simulink model "PIDnANNsim"  (R2021a)
settings: Solver=ode45  StartTime=0.0  StopTime=60  RelTol=1e-3  AbsTol=1e-6
undefined symbols (not defined in the file or in its folder): now, sfunxy2
libraries: neural x1, pid_lib x1
settings Model: ExtModeTrigMode=oneshot  ExtModeArmWhenConnect=off  TunableVars=prueba  TunableVarsStorageClass=Auto  Creator=The MathWorks, Inc.  LastModifiedBy=914487352
settings SolverCC: AutoScaleAbsTol=off  AlgebraicLoopSolver=TrustRegion
settings DataIOCC: SaveFormat=Array  SaveOutput=off  ReturnWorkspaceOutputs=off  SignalLoggingName=sigsOut
settings OptimizationCC: BooleanDataType=off  DefaultParameterBehavior=Inlined  ExpressionDepthLimit=2147483647  InitFltsAndDblsToZero=on  LifeSpan=inf
settings DebuggingCC: SaveWithParameterizedLinksMsg=none  UnderspecifiedInitializationDetection=Classic  MergeDetectMultiDrivingBlocksExec=none  SignalResolutionControl=TryResolveAllWithWarning  MultiTaskDSMMsg=warning  MultiTaskCondExecSysMsg=none  FcnCallInpInsideContextMsg=warning  StateNameClashWarn=warning  SFUnexpectedBacktrackingDiag=warning  SFNoUnconditionalDefaultTransitionDiag=warning  SFExecutionAtInitializationDiag=none  SFMachineParentedDataDiag=warning  ArithmeticOperatorsInVariantConditions=warning
settings HardwareCC: ProdBitPerPointer=32  ProdBitPerSizeT=32  ProdBitPerPtrDiffT=32  ProdLargestAtomicFloat=None  ProdIntDivRoundTo=Undefined  ProdEndianess=Unspecified  ProdWordSize=32  ProdHWDeviceType=32-bit Generic  TargetUnknown=on
settings ModelReferenceCC: PropagateSignalLabelsOutOfModel=off
settings SFSimCC: SimUseLocalCustomCode=off  CustomCodeUndefinedFunction=UseInterfaceOnly
settings RTWCC: TemplateMakefile=grt_vc.tmf  RTWUseLocalCustomCode=off
settings CodeAppCC: StateflowObjectComments=on
settings GRTTargetCC: TargetFcnLib=ansi_tfl_tmw.mat  TargetLangStandard=C89/C90 (ANSI)  CombineOutputUpdateFcns=off  GRTInterface=on
settings ConfigComp: CovMetricSettings=dw  CovSaveCumulativeToWorkspaceVar=on  CovSaveSingleToWorkspaceVar=on  CovExternalEMLEnable=off

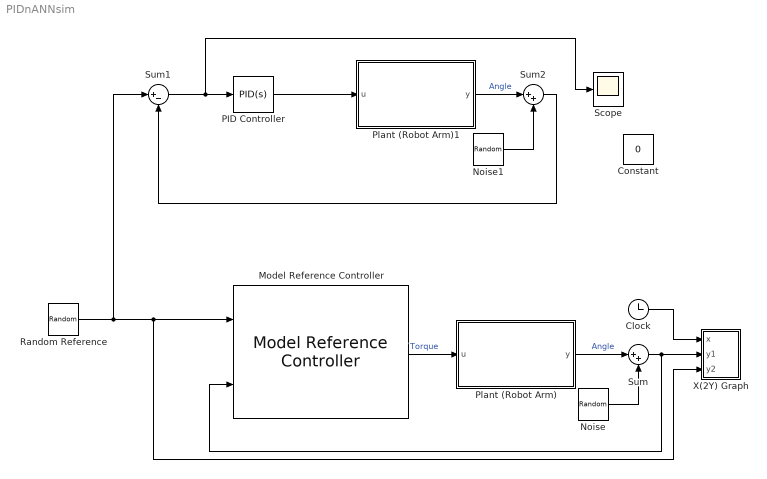
== system PIDnANNsim ==
  Clock : Clock
  Constant : Constant  Value=0
  Model Reference Controller : neural/Control Systems/Model Reference Controller  Nrc=2  Nic=1  Njc=2  IW_y=[0.15839265782647249381 0.22038419277684229147;0.20347680571023477047 -0.63453064159359129359;-1.4163043246094004779 -2.2531386406036326697;-2.4495799004731395598 -1.2012315278721505951;-0.18579754116155000609 -2.2638194953412376087;-1.8573874067270270682 0.06171935537830267049;-5.3645721606796019643 5.5441958314777801675;-0.98664431033243327196 -0.84730257551146492823;-1.0933287281864254581 0.49143784807095941547;-0.42041662548439218128 0.20871173651967303564]  IW_u=[-1.937141889835954478;-1.7914105891920755198;1.0113075975016061481;1.7405724858098692298;-0.23113891309024234277;-1.6474779127571286264;-0.013588487977038635549;2.1057052129704092458;0.98192223137069511996;0.26883521606040994278]  IW_r=[-5.3138547192394502972 -2.7684069091516758654;1.385878536939492145 1.6519866665000531025;-2.8750586159949764742 -3.5940790226772216798;-0.56304368137308291598 -0.65332618723348823142;1.7966096610782933407 -0.78020829833186511326;0.9664233503479621179 0.81952613480579372673;0.67011200103780099724 0.039371213727997830811;0.77003108717030610553 -1.1806545608518235202;-1.4046262152693724801 -1.0744787299127311897;0.88452426492441715844 -1.0427931854750644991]  B1_c=[-2.7370618367761849754;-1.0029353097437399001;-0.61844631303893637941;1.8907314655112790192;-0.040550822900097788226;-0.0001231396440501360864;-0.078786910253964809181;-0.69365557679911782341;-1.8127131460280845321;-1.8080439415409650383]  B2_c=1.241627577712959285  LW_c=[-3.2744750308658132631 1.9040971243521143119 -4.99897820247731417 -1.6704954268483922508 2.9763160613656429732 2.2387893177078401763 14.608154626501780982 -1.4444478720897002688 -1.4112785047422835571 1.6537064448285558882]  retraining_c=30  max_i_int=2  min_i_int=0.1  max_r_int=2  min_r_int=0.1  Ts=0.05  S1=10  Ni=2  Nj=2  sim_file=robotarm  trainfun=trainlm  Use_validation=1  Use_Testing=1  Use_Inc_training=0  Use_previous_weights=1  max_i=15  min_i=-15  max_r=0.7  min_r=-0.7  sam_training=10000  sam_training_c=6000  epochs=500  epochs_c=10  minp=-14.990217109796432737  maxp=14.944905782222949853  mint=-3.3174363789093801458  maxt=14.944905782222949853  Normalize=0  IW=[0.18683612490945086804 -0.29371364301366537086;-0.00029991909063309499543 -0.00030528826730701909796;0.00022130917238774274391 0.00019136116617624810885;-0.33113875798356290359 -0.1907051777282336158;-0.00011599472144967503979 -4.0589606688928513113e-05;-0.29964399912624584132 -0.012103654643994026657;0.13045830585147882852 -0.087708071898476264172;-0.00023311993864331110953 -0.00022351494184904346029;-0.00030337619752834177724 -0.00030093279833469268984;-0.38682124543143331374 0.23521510453583530098]  LW1_2=[0.57815072374799347799 0.40032181948406114769;-0.4734855345974983698 0.22508655222026188736;0.37300919718978625683 -0.16118707996705633478;-0.40934091798940658302 0.27351425234484955107;-0.4122207080899492615 0.069254034907186623471;0.93234837075850862664 -0.39719884612361677778;-0.0071613312115773415309 0.59186983238967516563;-0.40780350949764970769 0.17699535826217632772;-0.47393759565363408059 0.22446501232876728271;0.68764287837533344394 -0.22115389193832085679]  LW2_1=[-3.6884907355605128332e-05 -2.5819068720810176565 2.6618004759812468052 -4.7203617463710305913e-06 0.5728211564073127926 -2.0156117314578625084e-06 -3.9502160087481528832e-05 -1.1451273093513862911 -2.6381156452529261891 -2.6728299712317241135e-06]  B1=[-2.8878272681379240083;1.2702307200216940153;-0.096591249257216960089;0.78730941449699387569;0.0023422081542620494521;-0.33256389580091438862;1.0759814116288242136;-0.15889629203646479794;-1.2562597611588735003;2.4017885386895638788]  B2=0.036637277523094466392  S1c=10  Limit_output=1  min_output=-3.1  max_output=3.1  Ref_file=robotref
      settings: SourceProductBaseCode=NN
  Noise : UniformRandomNumber  Minimum=-0.5*0.1  Maximum=0.5*0.1  Seed=round(now)  SampleTime=10
  Noise1 : UniformRandomNumber  Minimum=-0.5*0.1  Maximum=0.5*0.1  Seed=round(now)  SampleTime=10
  PID Controller : pid_lib/PID Controller  Controller=PID  Form=Parallel  TimeDomain=Continuous-time  UseExternalTs=off  SampleTime=-1  IntegratorMethod=Forward Euler  FilterMethod=Forward Euler  ControllerParametersSource=internal  P=13.5094856642157  I=2.7058413528365  D=-4.58978335117057  UseFilter=on  N=100  TunerSelectOption=Transfer Function Based (PID Tuner App)  InitialConditionSource=internal  InitialConditionForIntegrator=0  InitialConditionForFilter=0  DifferentiatorICPrevScaledInput=0  ExternalReset=none  TrackingMode=off  Kt=1  LimitOutput=off  SatLimitsSource=internal  UpperSaturationLimit=inf  LowerSaturationLimit=-inf  LinearizeAsGain=on  AntiWindupMode=none  Kb=1  POutMin=[]  POutMax=[]  IOutMin=[]  IOutMax=[]  DOutMin=[]  DOutMax=[]  NOutMin=[]  NOutMax=[]  SumOutMin=[]  SumOutMax=[]  SaturationOutMin=[]  SaturationOutMax=[]  PParamMin=[]  PParamMax=[]  IParamMin=[]  IParamMax=[]  DParamMin=[]  DParamMax=[]  NParamMin=[]  NParamMax=[]  KbParamMin=[]  KbParamMax=[]  KtParamMin=[]  KtParamMax=[]  KbOutMin=[]  KbOutMax=[]  KtOutMin=[]  KtOutMax=[]  IntegratorOutMin=[]  IntegratorOutMax=[]  FilterOutMin=[]  FilterOutMax=[]  SumI1OutMin=[]  SumI1OutMax=[]  SumI2OutMin=[]  SumI2OutMax=[]  SumI3OutMin=[]  SumI3OutMax=[]  SumI4OutMin=[]  SumI4OutMax=[]  SumDOutMin=[]  SumDOutMax=[]  DifferentiatorOutMin=[]  DifferentiatorOutMax=[]  FilterDiffOutCoefMin=[]  FilterDiffOutCoefMax=[]  ReciprocalOutMin=[]  ReciprocalOutMax=[]  SumDenOutMin=[]  SumDenOutMax=[]  SumNumOutMin=[]  SumNumOutMax=[]  DivideOutMin=[]  DivideOutMax=[]  UdiffTsProdOutMin=[]  UdiffTsProdOutMax=[]  NTsProdOutMin=[]  NTsProdOutMax=[]  UintegralTsProdOutMin=[]  UintegralTsProdOutMax=[]  UngainTsProdOutMin=[]  UngainTsProdOutMax=[]  IntegratorContinuousStateAttributes=''  IntegratorStateMustResolveToSignalObject=off  IntegratorRTWStateStorageClass=Auto  FilterContinuousStateAttributes=''  FilterStateMustResolveToSignalObject=off  FilterRTWStateStorageClass=Auto  ParallelPVariant=InternalParameters  IdealPVariant=Disabled  IVariant=InternalParameters  DVariant=InternalParameters  IntegratorVariant=Continuous  SatVariant=Disabled  AWVariant=Passthrough  PCopyVariant=Disabled  TRVariant=Disabled  FdbkBlocksVariant=Forward  IdealPFdbkVariant=Disabled  SatFdbkVariant=Disabled  DerivativeFilterVariant=ContFilter  NVariant=InternalParameters  NCopyVariant=Disabled  FilterICVariant=InternalICsFilter  IntegratorICVariant=InternalICs  ExternalResetVariant=Disabled  TRSumVariant=Passthrough  SumFdbkVariant=Disabled  SumVariant=Sum_PID  TsampFilterVariant=InternalTs  TsampNgainVariant=Passthrough  TsampIntegralVariant=Passthrough  ExternalSaturationOutDataTypeStr=Inherit: Same as second input
  Plant (Robot Arm) : Subsystem
      mask Display: plot([-10],[0],[10],[0],[-2 -2 2 2 -2],[5 4 4 5 5],[0 3],[4.5 0.5])
  Plant (Robot Arm)1 : Subsystem
      mask Display: plot([-10],[0],[10],[0],[-2 -2 2 2 -2],[5 4 4 5 5],[0 3],[4.5 0.5])
  Random Reference : UniformRandomNumber  Minimum=-0.5  Maximum=0.5  Seed=round(now)  SampleTime=10
  Scope : Scope
  Sum : Sum  Inputs=|++
  Sum1 : Sum  Inputs=|+-
  Sum2 : Sum  Inputs=|++
  X(2Y) Graph : Subsystem  LoadFcn=sfunxy2([],[],[],'LoadBlock')  StartFcn=sfunxy2([],[],[],'Start')  StopFcn=sfunxy2([],[],[],'Stop')  mask(X(2Y) scope.){xmin=0, xmax=5, ymin=-1, ymax=1, st=-1}
      mask prompts: xmin "x-min:"; xmax "x-max:"; ymin "y-min:"; ymax "y-max:"; st "Sample time:"
      mask help: X(2Y) scope using MATLAB graph window. First input is used as time base. Enter plotting ranges.
      settings: CopyFcn=sfunxy2([],[],[],'CopyBlock')  DeleteFcn=sfunxy2([],[],[],'DeleteBlock')  NameChangeFcn=sfunxy2([],[],[],'NameChange')
      mask Help: This block can be used to explore limit cycles. Look at the function sfunxy.m to see how it works.
      mask Display: plot([.05 .95 .95 .05 .05],[.45 .45 .95 .95 .45], 0.5+cos(0:0.1:2*pi)*0.3,0.7+sin(0:0.1:2*pi)*0.2)
  wires:
  Model Reference Controller/1 -> Plant (Robot Arm)/1(u)  "Torque"
  Clock/1 -> X(2Y) Graph/1(x)
  Random Reference/1 -> Sum1/1, X(2Y) Graph/3(y2), Model Reference Controller/1
  Plant (Robot Arm)/1(y) -> Sum/1  "Angle"
  Sum/1 -> X(2Y) Graph/2(y1), Model Reference Controller/2
  Sum1/1 -> Scope/1, PID Controller/1
  PID Controller/1 -> Plant (Robot Arm)1/1(u)
  Sum2/1 -> Sum1/2
  Plant (Robot Arm)1/1(y) -> Sum2/1  "Angle"
  Noise/1 -> Sum/2
  Noise1/1 -> Sum2/2

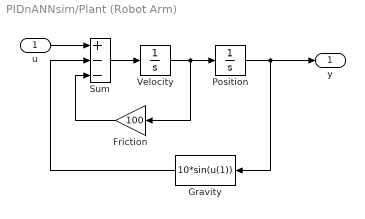
== system PIDnANNsim/Plant (Robot Arm) ==
  u : Inport
  Friction : Gain  Gain=100  SaturateOnIntegerOverflow=on  OutDataTypeStr=Inherit: Same as input  ParamDataTypeStr=Inherit: Same as input
  Gravity : Fcn  Expr=10*sin(u(1))
  Position : Integrator  ZeroCross=off
  Sum : Sum  Inputs=+--  InputSameDT=on  SaturateOnIntegerOverflow=on  OutDataTypeStr=Inherit: Same as first input
  Velocity : Integrator  ZeroCross=off
  y : Outport
  wires:
  Position/1 -> y/1, Gravity/1
  u/1 -> Sum/1
  Sum/1 -> Velocity/1
  Gravity/1 -> Sum/2
  Velocity/1 -> Position/1, Friction/1
  Friction/1 -> Sum/3

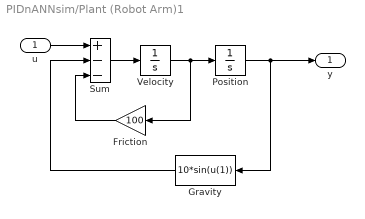
== system PIDnANNsim/Plant (Robot Arm)1 ==
  u : Inport
  Friction : Gain  Gain=100  SaturateOnIntegerOverflow=on  OutDataTypeStr=Inherit: Same as input  ParamDataTypeStr=Inherit: Same as input
  Gravity : Fcn  Expr=10*sin(u(1))
  Position : Integrator  ZeroCross=off
  Sum : Sum  Inputs=+--  InputSameDT=on  SaturateOnIntegerOverflow=on  OutDataTypeStr=Inherit: Same as first input
  Velocity : Integrator  ZeroCross=off
  y : Outport
  wires:
  Position/1 -> y/1, Gravity/1
  u/1 -> Sum/1
  Sum/1 -> Velocity/1
  Gravity/1 -> Sum/2
  Velocity/1 -> Position/1, Friction/1
  Friction/1 -> Sum/3

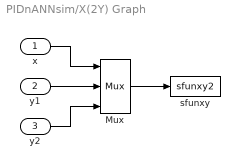
== system PIDnANNsim/X(2Y) Graph ==
  x : Inport
  y1 : Inport  Port=2
  y2 : Inport  Port=3
  Mux : Mux  Inputs=3
  sfunxy : S-Function  FunctionName=sfunxy2  Parameters=[xmin xmax ymin ymax], st  SFunctionDeploymentMode=off  EnableBusSupport=off
  wires:
  y2/1 -> Mux/3
  y1/1 -> Mux/2
  x/1 -> Mux/1
  Mux/1 -> sfunxy/1
